simulink model "Powertrain_ECU_SIL"  (R2026a)
settings: Solver=FixedStepAuto  StopTime=50  MaxStep=0.001  MinStep=0.0001  AbsTol=1e-6
InitFcn:
  | run('Vehicle_parameters_values_V1_MIL.m')
libraries: slpidlib x1
settings Model: PacingRate=0.500000  Creator=irfan  LastModifiedBy=irfan
settings SolverCC: ShapePreserveControl=EnableAll  ZeroCrossControl=EnableAll  ZeroCrossAlgorithm=Adaptive  MinimalZcImpactIntegration=on
settings DebuggingCC: ReadBeforeWriteMsg=DisableAll  WriteAfterWriteMsg=DisableAll  WriteAfterReadMsg=DisableAll  MultiTaskDSMMsg=none
settings SFSimCC: SFSimEcho=off
settings RTWCC: SystemTargetFile=ert.tlc  Description=Embedded Coder
settings ERTTargetCC: GenerateSampleERTMain=on  SupportContinuousTime=on

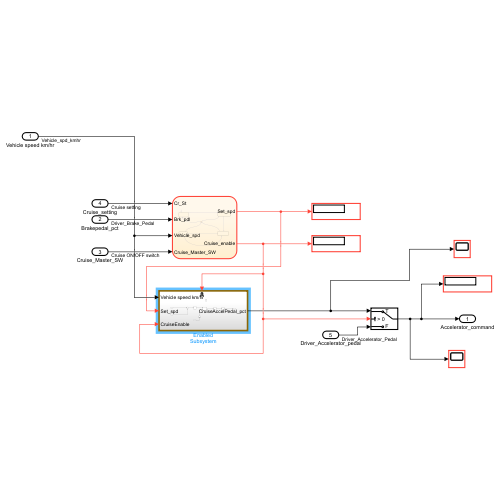
[thumbnail: Simulink's stored preview of the top-level diagram]
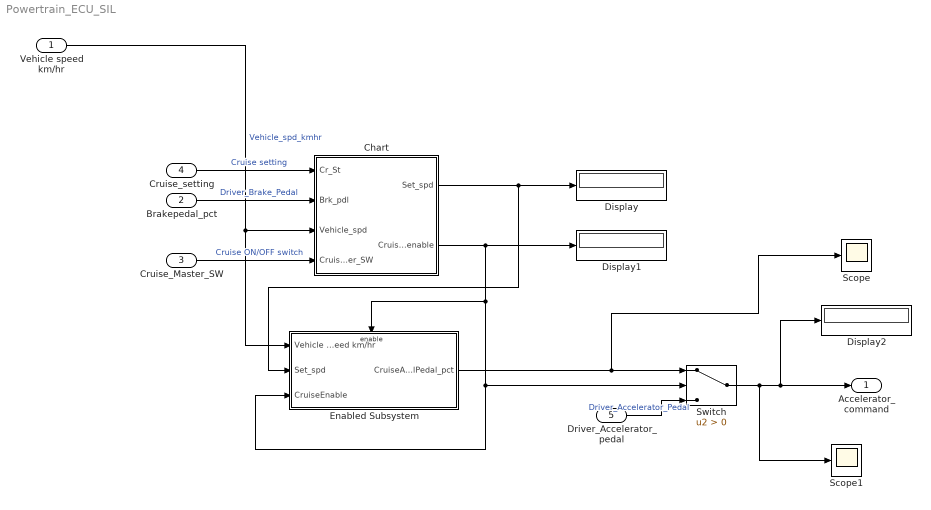
== system Powertrain_ECU_SIL ==
  Vehicle speed km/hr : Inport  OutDataTypeStr=double  PortDimensions=1
  Brakepedal_pct : Inport  Port=2  OutDataTypeStr=double  PortDimensions=1
  Cruise_Master_SW : Inport  Port=3  OutDataTypeStr=double  PortDimensions=1
  Cruise_setting : Inport  Port=4  OutDataTypeStr=double  PortDimensions=1
  Driver_Accelerator_pedal : Inport  Port=5  OutDataTypeStr=double  PortDimensions=1
  Chart : Stateflow chart  TreatAsAtomicUnit=on
  Display : Display
  Display1 : Display
  Display2 : Display
  Enabled Subsystem : Subsystem  TreatAsAtomicUnit=on
  Scope : Scope
      settings: ActiveDisplayYMinimum=-1  ActiveDisplayYMaximum=1  DataLoggingVariableName=ScopeData6
  Scope1 : Scope
      settings: ActiveDisplayYMinimum=-5.6388294949677089  ActiveDisplayYMaximum=36.997696709911374  DataLoggingVariableName=ScopeData7
  Switch : Switch  Criteria=u2 > Threshold  SaturateOnIntegerOverflow=off  InputSameDT=off
  Accelerator_command : Outport  OutDataTypeStr=double  PortDimensions=1
  wires:
  Chart/1(Set_spd) -> Display/1, Enabled Subsystem/2(Set_spd)
  Vehicle speed km/hr/1 -> Enabled Subsystem/1(Vehicle speed km/hr), Chart/3(Vehicle_spd)  "Vehicle_spd_kmhr"
  Cruise_Master_SW/1 -> Chart/4(Cruise_Master_SW)  "Cruise ON/OFF switch"
  Brakepedal_pct/1 -> Chart/2(Brk_pdl)  "Driver_Brake_Pedal"
  Enabled Subsystem/1(CruiseAccelPedal_pct) -> Switch/1, Scope/1
  Cruise_setting/1 -> Chart/1(Cr_St)  "Cruise setting"
  Chart/2(Cruise_enable) -> Switch/2, Enabled Subsystem/3(CruiseEnable), Enabled Subsystem/Enable, Display1/1
  Driver_Accelerator_pedal/1 -> Switch/3  "Driver_Accelerator_Pedal"
  Switch/1 -> Accelerator_command/1, Display2/1, Scope1/1

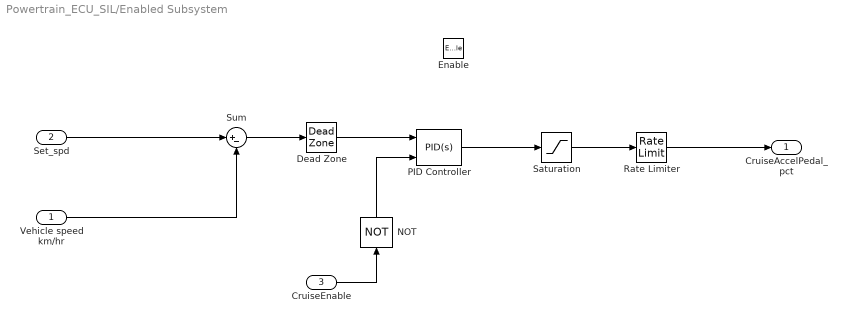
== system Powertrain_ECU_SIL/Enabled Subsystem ==
  Vehicle speed km/hr : Inport
  Set_spd : Inport  Port=2
  CruiseEnable : Inport  Port=3
  Enable : EnablePort  StatesWhenEnabling=reset
  Dead Zone : DeadZone
  NOT : Logic  Operator=NOT  IconShape=distinctive  AllPortsSameDT=off  OutDataTypeStr=boolean
  PID Controller : slpidlib/PID Controller  Controller=PID  Form=Parallel  TimeDomain=Continuous-time  UseExternalTs=off  SampleTime=-1  IntegratorMethod=Forward Euler  FilterMethod=Forward Euler  ControllerParametersSource=internal  P=1  I=0.5  UseKiTs=off  D=0  UseExternalDerivativeSource=off  N=100  UseFilter=on  TunerSelectOption=Transfer Function Based (PID Tuner App)  InitialConditionSource=internal  InitialConditionForIntegrator=0  InitialConditionForFilter=0  DifferentiatorICPrevScaledInput=0  ExternalReset=rising  TrackingMode=off  Kt=1  LimitOutput=on  SatLimitsSource=internal  UpperSaturationLimit=100  LowerSaturationLimit=0  LinearizeAsGain=on  AntiWindupMode=back-calculation  Kb=1  LimitIntegrator=off  UpperIntegratorSaturationLimit=inf  LowerIntegratorSaturationLimit=-inf  POutMin=[]  POutMax=[]  IOutMin=[]  IOutMax=[]  DOutMin=[]  DOutMax=[]  NOutMin=[]  NOutMax=[]  SumOutMin=[]  SumOutMax=[]  SaturationOutMin=[]  SaturationOutMax=[]  PParamMin=[]  PParamMax=[]  IParamMin=[]  IParamMax=[]  DParamMin=[]  DParamMax=[]  NParamMin=[]  NParamMax=[]  KbParamMin=[]  KbParamMax=[]  KtParamMin=[]  KtParamMax=[]  KbOutMin=[]  KbOutMax=[]  KtOutMin=[]  KtOutMax=[]  IntegratorOutMin=[]  IntegratorOutMax=[]  FilterOutMin=[]  FilterOutMax=[]  SumI1OutMin=[]  SumI1OutMax=[]  SumI2OutMin=[]  SumI2OutMax=[]  SumI3OutMin=[]  SumI3OutMax=[]  SumI4OutMin=[]  SumI4OutMax=[]  SumDOutMin=[]  SumDOutMax=[]  DifferentiatorOutMin=[]  DifferentiatorOutMax=[]  FilterDiffOutCoefMin=[]  FilterDiffOutCoefMax=[]  ReciprocalOutMin=[]  ReciprocalOutMax=[]  SumDenOutMin=[]  SumDenOutMax=[]  SumNumOutMin=[]  SumNumOutMax=[]  DivideOutMin=[]  DivideOutMax=[]  UdiffTsProdOutMin=[]  UdiffTsProdOutMax=[]  NTsProdOutMin=[]  NTsProdOutMax=[]  UintegralTsProdOutMin=[]  UintegralTsProdOutMax=[]  UngainTsProdOutMin=[]  UngainTsProdOutMax=[]  ClampingZeroOutDataTypeStr=Inherit: Inherit via back propagation  ClampingZeroOutMin=[]  ClampingZeroOutMax=[]  FilterDenConstantOutDataTypeStr=Inherit: Inherit via back propagation  FilterDenConstantOutMin=[]  FilterDenConstantOutMax=[]  PCopyOutDataTypeStr=Inherit: Inherit via back propagation  PCopyOutMin=[]  PCopyOutMax=[]  NCopyOutDataTypeStr=Inherit: Inherit via back propagation  NCopyOutMin=[]  NCopyOutMax=[]  IntegratorContinuousStateAttributes=''  IntegratorStateMustResolveToSignalObject=off  IntegratorRTWStateStorageClass=Auto  FilterContinuousStateAttributes=''  FilterStateMustResolveToSignalObject=off  FilterRTWStateStorageClass=Auto  ParallelPVariant=InternalParameters  IdealPVariant=Disabled  IVariant=InternalParameters  DVariant=InternalParameters  IntegratorVariant=Continuous  SatVariant=Enabled  AWVariant=BackCalculation  PCopyVariant=Disabled  TRVariant=Disabled  FdbkBlocksVariant=Forward  IdealPFdbkVariant=Disabled  SatFdbkVariant=Disabled  DerivativeFilterVariant=ContFilter  NVariant=InternalParameters  NCopyVariant=Disabled  FilterICVariant=InternalICsFilter  IntegratorICVariant=InternalICs  ExternalResetVariant=ExternalReset  TRSumVariant=Passthrough  SumFdbkVariant=Disabled  SumVariant=Sum_PID  TsampFilterVariant=InternalTs  TsampNgainVariant=Passthrough  TsampIntegralVariant=Disabled_SignalSpec  ExternalSaturationOutDataTypeStr=Inherit: Same as second input  DerivativeSourceVariant=ErrorSignal  PreIntVariant=InternalPreInt
  Rate Limiter : RateLimiter  RisingSlewLimit=25  FallingSlewLimit=-40  SampleTimeMode=inherited
  Saturation : Saturate  UpperLimit=100  LowerLimit=0
  Sum : Sum  Inputs=|+-
  CruiseAccelPedal_pct : Outport
  wires:
  Dead Zone/1 -> PID Controller/1
  Rate Limiter/1 -> CruiseAccelPedal_pct/1
  PID Controller/1 -> Saturation/1
  Set_spd/1 -> Sum/1
  Vehicle speed km/hr/1 -> Sum/2
  NOT/1 -> PID Controller/2
  CruiseEnable/1 -> NOT/1
  Saturation/1 -> Rate Limiter/1
  Sum/1 -> Dead Zone/1

== stateflow chart Powertrain_ECU_SIL/Chart ==
  state READY
    entry:
    Set_spd = Vehicle_spd;
    Cruise_enable=0;
  state OFF
    during:
    Cruise_enable=0;
  state ACTIVE
    during:
    Cruise_enable=1;
  state STANDBY
    during:
    Cruise_enable=0;
  (default) -> OFF
  OFF -> READY : [Cruise_Master_SW==1 && Cr_St==1 && Vehicle_spd>MinCruiseSpd]
  READY -> (junction 19) [order 2]
  READY -> ACTIVE [order 1] : [true]
  (junction 19) -> OFF : [Cruise_Master_SW==0]
  ACTIVE -> (junction 19) [order 2]
  STANDBY -> (junction 19) [order 2]
  ACTIVE -> STANDBY [order 1] : [Cruise_Master_SW==1 && Cr_St==0 || Brk_pdl>0]
  STANDBY -> ACTIVE [order 1] : [Cruise_Master_SW==1 && Cr_St==2]
  data: Cr_St input; Brk_pdl input; Set_spd output; Cruise_enable output; Vehicle_spd input; MinCruiseSpd parameter; Cruise_Master_SW input
